simulink model "CustomSliders"  (R2025b)
settings: Solver=VariableStepAuto  StartTime=0.0  StopTime=10.0  RelTol=1e-3
settings Model: PacingRate=0.800000  Creator=The MathWorks, Inc.  LastModifiedBy=gkumares
settings OptimizationCC: ReuseModelBlockBuffer=off
settings RTWCC: GPUComputeCapability=3.5

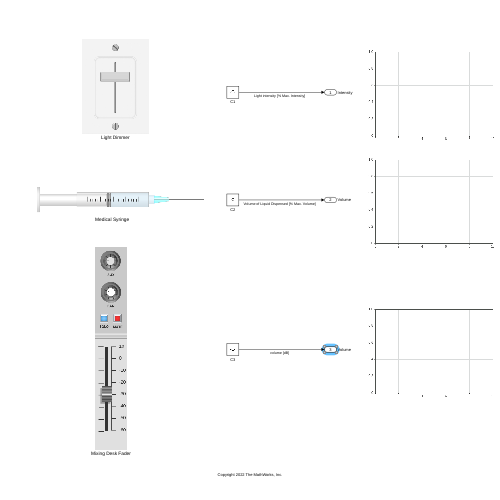
[thumbnail: Simulink's stored preview of the top-level diagram]
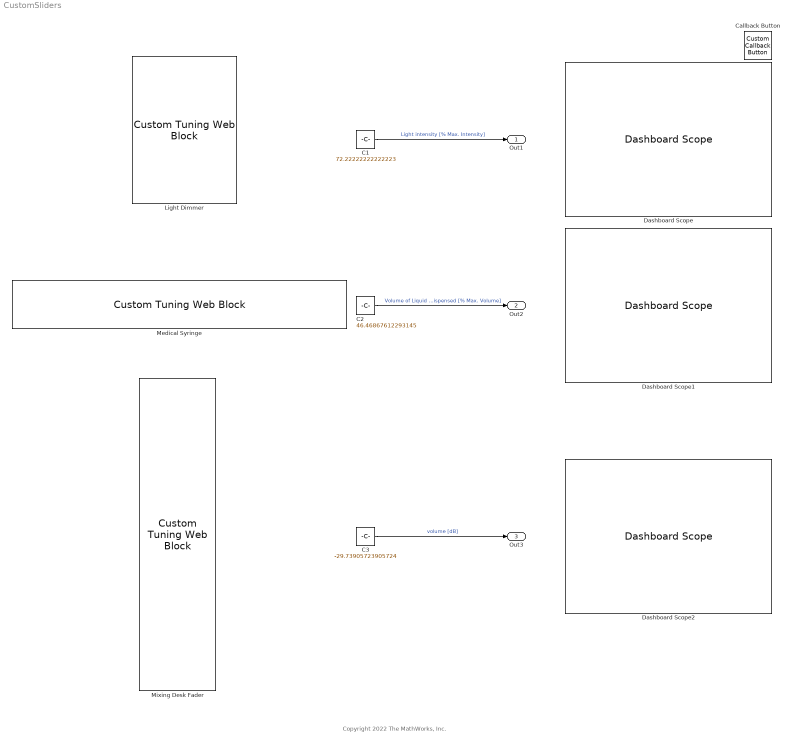
== system CustomSliders ==
  note: Copyright 2022 The MathWorks, Inc.
  C1 : Constant  Value=72.22222222222223
  C2 : Constant  Value=46.46867612293145
  C3 : Constant  Value=-29.73905723905724
  Callback Button : CustomCallbackButton  Configuration="{\"components\":[{\"name\":\"BackgroundImageComponent\",\"settings\":{\"image\":{\"size\":[0,0],\"src\":\"default\",\"srcOrientation\":\"Right\"},\"position\":[0,0,1,1]}},{\"name\":\"ButtonStateComponent\",\"settings\":{\"buttonType\":\"momentary\",\"clickFcn\":\"showExample('simulink\\/DesignCustomSlidersExample');\",\"onValue\":1,\"position\":[0,0,1,1],\"pressDelay\":\"500\",\"pressFcn\":\"\",\"repeatInterval\":\"0\",\"states\":[{\"horizontalAlignment\":\"center\",\"image\":{\"position\":[0,0,1,1],\"src\":\"default\",\"srcOrientation\":\"Right\"},\"label\":{\"color\":[0.01176470588,0.01176470588,0.01176470588,1],\"icon\":{\"size\":[0,0],\"src\":\"default\",\"srcOrientation\":\"Right\"},\"iconPlacement\":\"left\",\"text\":{\"content\":\"?\"}},\"labelOffset\":[0,0],\"verticalAlignment\":\"middle\"},{\"horizontalAlignment\":\"center\",\"image\":{\"position\":[0,0,1,1],\"src\":\"default\",\"srcOrientation\":\"Right\"},\"label\":{\"color\":[0.01176470588,0.01176470588,0.01176470588,1],\"icon\":{\"size\":[0,0],\"src\":\"default\",\"srcOrientation\":\"Right\"},\"iconPlacement\":\"left\",\"text\":{\"content\":\"?\"}},\"labelOffset\":[0,0],\"verticalAlignment\":\"middle\"},{\"horizontalAlignment\":\"center\",\"image\":{\"position\":[0,0,1,1],\"src\":\"default\",\"srcOrientation\":\"Right\"},\"label\":{\"color\":[0.01176470588,0.01176470588,0.01176470588,1],\"icon\":{\"size\":[0,0],\"src\":\"default\",\"srcOrientation\":\"Right\"},\"iconPlacement\":\"left\",\"text\":{\"content\":\"?\"}},\"labelOffset\":[0,0],\"verticalAlignment\":\"middle\"},{\"horizontalAlignment\":\"center\",\"image\":{\"position\":[0,0,1,1],\"src\":\"default\",\"srcOrientation\":\"Right\"},\"label\":{\"color\":[0.01176470588,0.01176470588,0.01176470588,1],\"icon\":{\"size\":[0,0],\"src\":\"default\",\"srcOrientation\":\"Right\"},\"iconPlacement\":\"left\",\"text\":{\"content\":\"?\"}},\"labelOffset\":[0,0],\"verticalAlignment\":\"middle\"}]}},{\"name\":\"ForegroundImageComponent\",\"settings\":{\"image\":{\"size\":[0,0],\"src\":\"default\",\"srcOrientation\":\"Right\"},\"isForeground\":1,\"position\":[0,0,1,1]}}],\"derived\":{\"blockParameters\":{\"AutoActivate\":true,\"ButtonText\":\"?\",\"ButtonType\":\"Momentary\",\"ClickFcn\":\"showExample('simulink\\/DesignCustomSlidersExample');\",\"OnValue\":1,\"PressDelay\":\"500\",\"PressFcn\":\"\",\"RepeatInterval\":\"0\",\"fixedAspectRatio\":\"off\"}},\"settings\":{\"BindingType\":\"standalone\",\"autoActivate\":true,\"backgroundColor\":[244,244,244,1],\"backgroundOffset\":0.2,\"backgroundOpacity\":1,\"fixedAspectRatio\":\"off\",\"foregroundColor\":[0.01176470588,0.01176470588,0.01176470588,1],\"migratedFromLegacy\":true,\"useBackgroundColor\":true,\"variant\":\"callback\",\"version\":\"R2025a\"},\"type\":\"Button\"}"  CustomBackgroundColor="{\"color\":[0.9568627451,0.9568627451,0.9568627451],\"show\":true}"
  Dashboard Scope : DashboardScope  Ymin=0  Ymax=1  FontColor=[0.0, 0.0, 0.0]
  Dashboard Scope1 : DashboardScope  Ymin=0  Ymax=1  FontColor=[0.0, 0.0, 0.0]
  Dashboard Scope2 : DashboardScope  Ymin=0  Ymax=1  FontColor=[0.0, 0.0, 0.0]
  Light Dimmer : CustomTuningWebBlock  LabelPosition=Hide  ShowInitialText=on  Configuration="{\"components\":[{\"name\":\"LinearScaleComponent\",\"settings\":{\"bounds\":{\"max\":100,\"min\":0,\"tickInterval\":\"auto\"},\"internalTickHeightScaleFactor\":0.5,\"labelColor\":[255,255,200],\"labelFont\":{\"font\":\"Arial\",\"fontSize\":12},\"labelOffset\":0.05,\"labelTransparency\":1,\"needleImage\":{\"size\":[1144,1604],\"src\":\"data:image\\/png;base64,iVBORw0KGgoAAAANSUhEUgAABHgAAAZECAYAAACZ1be8AAAAAXNSR0IArs4c6QAAAARnQU1BAACxjwv8YQUAAAAJcEhZcwAAMsAAADLAAShkWtsAADEiSURBVHhe7d35s9d13f\\/x\\/oGmbWqmnMpSy7AwM8usAM3UzA1cisIFM1EDAY0QBQ+LiiKCLFqAcBb2TZBN9gMKxL64gNLUKWumsn6pZrKpptfF83Wdz7mw8Opc+Xm\\/r4+H223mPhD1vX79fL6Pz+v9er8NAAAAAAAAAAAAAAAAAAAAAAAAAAAAAAAAAAAAAAAAAAAAAAAAAAAAAAAAAAAAAAAAAAAAAAAAAAAAAAAAAAAAAAAAAAAAAAAAAAAAAAAAAAAAAAAAAAAAAAAAAAAAAA ...(+16878 chars)\",\"srcOrientation\":\"Up\"},\"needleOffset\":[0.004661239495798319,-0.48886434750598196],\"needleSize\":{\"height\":1,\"width\":1},\"position\":[0.21691176470588236,0.44202098288238545,0.4734032762746181,0.5877100840336135],\"referencePoint\":\"auto\",\"scaleColors\":[],\"scaleColorsSize\":0.2,\"scaleDirection\":\"BT\",\"showLabels\":false,\"showMinorTicks\":0,\"showSpanLine\":false,\"showTicks\":false,\"tickColor\":[0,0,0],\"tickTransparency\":1,\"valueBarColor\":[0,114,189],\"valueBarOffset\":-0.27,\"valueBarSize\":0.1,\"valueBarTransparency\":0}},{\"name\":\"BackgroundImageComponent\",\"settings\":{\"image\":{\"size\":[1145,1605],\"src\":\"data:image\\/png;base64,iVBORw0KGgoAAAANSUhEUgAABHkAAAZFCAMAAACKlf8VAAAAAXNSR0IArs4c6QAAAARnQU1BAACxjwv8YQUAAAKUUExURdnZ2fLy8ubm5s3NzcHBwba2tqqqqp6enpKSkpGRkZqamqenp6WlpbKysq+vr729vbu7u8jIyOTk5Nra2q2traSkpKOjo6ampqioqKmpqaKiop+fn52dnZubm5iYmJOTk42NjYaGhri4uMXFxePj46ysrLCwsLOzs7Gxsa6urqurq6CgoJSUlI6OjsPDw6GhobS0tLW1tbe3t7m5ubq6upeXl4SEhImJieLi4ry8vL6+vr+\\/v8DAwIqKin9\\/f+Hh4cTExMLCwsbGxsfHx8nJycrKypycnJmZmZaWloKCgnNzc+Dg ...(+380064 chars)\",\"srcOrientation\":\"Up\"},\"position\":[0,0,1,1],\"scaleMode\":\"0\"}},{\"name\":\"ForegroundImageComponent\",\"settings\":{\"image\":{\"size\":[0,0],\"src\":\"default\",\"srcOrientation\":[]},\"isForeground\":1,\"position\":[0,0,1,1],\"scaleMode\":\"0\"}}],\"derived\":{\"blockParameters\":{\"ForegroundColor\":[0,0,0],\"Limits\":{\"Max\":100,\"Min\":0,\"Ticks\":\"auto\"},\"ScaleColors\":[],\"ScaleDirection\":\"Clockwise\",\"ScaleMax\":100,\"ScaleMin\":0,\"TickInterval\":\"auto\",\"fixedAspectRatio\":\"on\"}},\"settings\":{\"BindingType\":\"param\",\"aspectRatio\":3.7777777777777777,\"backgroundColor\":[0,0,0,\"1\"],\"backgroundOffset\":0,\"backgroundOpacity\":1,\"fixedAspectRatio\":\"on\",\"foregroundColor\":[252,252,196],\"orientation\":\"vertical\",\"showBackgroundColor\":false,\"value\":0,\"version\":\"R2023a\"},\"type\":\"LinearGauge\"}"
  Medical Syringe : CustomTuningWebBlock  LabelPosition=Hide  ShowInitialText=on  Configuration="{\"components\":[{\"name\":\"LinearScaleComponent\",\"settings\":{\"bounds\":{\"max\":100,\"min\":0,\"tickInterval\":\"auto\"},\"internalTickHeightScaleFactor\":0.5,\"labelColor\":[255,255,200],\"labelFont\":{\"font\":\"Arial\",\"fontSize\":12},\"labelOffset\":0.05,\"labelTransparency\":1,\"needleImage\":{\"size\":[2348,344],\"src\":\"data:image\\/png;base64,iVBORw0KGgoAAAANSUhEUgAACSwAAAFYCAMAAABk09DVAAAAAXNSR0IArs4c6QAAAARnQU1BAACxjwv8YQUAAAG\\/UExURQAAALbl\\/wAAAAQEBAcHBwgICAsLCwwMDA4ODhAQEBERERQUFBgYGBsbGx4eHh8fHyEhISMjIyQkJCYmJicnJykpKSoqKiwsLC0tLTAwMDMzMzY2Njc3Nzg4ODo6Ojs7Oz09PUBAQEJCQkNDQ0VFRUZGRkdHR0lJSUtLS0xMTE5OTlBQUFFRUVJSUlNTU1RUVFZWVlhYWFlZWVpaWltbW11dXV9fX2FhYWJiYmNjY2RkZGZmZmdnZ2lpaWpqamtra2xsbG1tbW5ubm9vb3BwcHFxcXJycnNzc3R0dHV1dXZ2dnd3 ...(+5320 chars)\",\"srcOrientation\":\"Right\"},\"needleOffset\":[-0.10051546391752578,-0.004172421731123388],\"needleSize\":{\"height\":1,\"width\":1},\"position\":[0.01885680612846199,0.3773020257826888,0.26033034069981587,0.973089766254174],\"referencePoint\":\"auto\",\"scaleColors\":[],\"scaleColorsSize\":0.2,\"scaleDirection\":\"LR\",\"showLabels\":false,\"showMinorTicks\":0,\"showSpanLine\":false,\"showTicks\":false,\"tickColor\":[0,0,0],\"tickTransparency\":1,\"valueBarColor\":[0,114,189],\"valueBarOffset\":-0.27,\"valueBarSize\":0.1,\"valueBarTransparency\":0}},{\"name\":\"BackgroundImageComponent\",\"settings\":{\"image\":{\"size\":[2348,344],\"src\":\"data:image\\/png;base64,iVBORw0KGgoAAAANSUhEUgAACSwAAAFYCAMAAABk09DVAAAAAXNSR0IArs4c6QAAAARnQU1BAACxjwv8YQUAAAAGUExURf\\/\\/\\/wAAAFXC034AAAACdFJOU\\/8A5bcwSgAAAAlwSFlzAAAywAAAMsABKGRa2wAAAyVJREFUeF7twQEBAAAAgiD\\/r25IQAAAAAAAAAAAAAAAAAAAAAAAAAAAAAAAAAAAAAAAAAAAAAAAAAAAAAAAAAAAAAAAAAAAAAAAAAAAAAAAAAAAAAAAAAAAAAAAAAAAAAAAAAAAAAAAAAAAAAAAAAAAAAAAAAAAAAAAAAAAAAAAAAAAAAAAAAAAAAAAAAAAAAAAAAAAAAAAAAAAAAAAAAAAAAAAAAAAAAAAAAAAAAAAAAAAAAAAAAAAAAAAAAAAAAAAAAAAAAAAAAAAAAAAAAAAAAAAAAAAAAAAAAAAAAAAAAAAAAAAAAAAAAAAAAAAAAAAAAAAAAAAAAAAAAAAAAAAAAAAAAAAAAAAAAAAAAAAAAAAAAAAAAAAAAAAAAAAAAAAAAAAAAAAAAAAAAAAAAAAAAAAAAAAAAAAAAAAAAAAAAAAAAAAAAAAAAAAAAAAAAAAAAAAAAAAAAAAAAAAAAAAAAAAAAAAAAAAAAAAAAAAAAAAAAAAAAAAAAAAAAAAAAAAAAAAAAAAAAAAAAAAAAAAAAAAAAAAAAAAAAAAAAAAAAAAAAAAAAAAAAAAAAAAAAAAAAAAAAAAAAAAAAAAAAAAAAAAAAAAAAAAAAAAAAAAAAAAAAAAAAAAAAAAAAAAAAAAAAAAAAAAAAAAAAAAAAAAAAAAAAAAAAAAAAAAAAAAAAAAAAAAAAAAAAAAAAAAAAAAAAAAAAAAAAAAAAAAAAAAAAAAAAAAAAAAAAAAAAAAAAAAAAAAAAAAAAAAAAAAAAAAAAAAAAAAAAAAAAAAAAAAAAAAAAAAAAAAAAAAAAAAAAAAAAAAAAAAAAAAAAAAAAAAAAAAAAAAAAAAAAAAAAAAAAAAAAAAAAAAAAAAAAAAAAAAAAAAAAAAAAAAAAAAAAAAAAAAAAAAAAAAAAAAAAAAAAAAAAAAAAAAAAAAAAAAAAAAAAAAAAAAAAAAAAAAAAAAAAAAAAAAAAAAAAAAAAAAAAAAAAAAAAAAAAAAAAAAAAAAAAAAAAAAAAAAAAAAAAAAAAAAAAAAAAAAAAAAAAAAAAAAAAAAAAAAAAAAAAAAAAAAwLkaVSwAAQ05s70AAAAASUVORK5CYII=\",\"srcOrientation\":\"Right\"},\"position\":[0,0,1,1],\"scaleMode\":\"0\"}},{\"name\":\"ForegroundImageComponent\",\"settings\":{\"angle\":0,\"image\":{\"size\":[2348,344],\"src\":\"data:image\\/png;base64,iVBORw0KGgoAAAANSUhEUgAACSwAAAFYCAYAAABTDSDnAAAAAXNSR0IArs4c6QAAAARnQU1BAACxjwv8YQUAAAAJcEhZcwAAMsAAADLAAShkWtsAADmMSURBVHhe7d3Lr271nef3Uv8LPahRS51ZR1EPMkikTNKtZJRJRVYGUalqUKNuKRlE6o6UKBXZD5wrHC7masAGcylsc\\/EFMBgHzB0frjZ3MMdwDBjDMcXdGOOjvX95nu31xe3sjx9Xzm9vs9Zer5f0lqqsr89X+FmDtc7vV66\\/AAAAAAAAAAAAAAAAAAAAAAAAAAAAAAAAAAAAAAAAAAAAAAAAAAAAAAAAAAAAAAAAAAAAAAAAAAAAAAAAAAAAAAAAAAAAAAAAAAAAAAAAAAAAAAAA ...(+20020 chars)\"},\"isForeground\":1,\"position\":[0,0.0017840699815837937,1,1],\"scaleMode\":\"0\"}}],\"derived\":{\"blockParameters\":{\"ForegroundColor\":[0,0,0],\"Limits\":{\"Max\":100,\"Min\":0,\"Ticks\":\"auto\"},\"ScaleColors\":[],\"ScaleDirection\":\"Clockwise\",\"ScaleMax\":100,\"ScaleMin\":0,\"TickInterval\":\"auto\",\"fixedAspectRatio\":\"on\"}},\"settings\":{\"BindingType\":\"param\",\"aspectRatio\":3.7777777777777777,\"backgroundColor\":[0,0,0,\"1\"],\"backgroundOffset\":0,\"backgroundOpacity\":1,\"fixedAspectRatio\":\"on\",\"foregroundColor\":[252,252,196],\"orientation\":\"horizontal\",\"showBackgroundColor\":false,\"value\":0,\"version\":\"R2023a\"},\"type\":\"LinearGauge\"}"
  Mixing Desk Fader : CustomTuningWebBlock  LabelPosition=Hide  ShowInitialText=on  Configuration="{\"components\":[{\"name\":\"LinearScaleComponent\",\"settings\":{\"bounds\":{\"max\":10,\"min\":-60,\"tickInterval\":\"auto\"},\"internalTickHeightScaleFactor\":1,\"labelColor\":[0,0,0],\"labelFont\":{\"font\":\"Arial\",\"fontSize\":12},\"labelOffset\":0.15,\"labelTransparency\":1,\"needleImage\":{\"size\":[97,144],\"src\":\"data:image\\/png;base64,iVBORw0KGgoAAAANSUhEUgAAAGEAAACQCAMAAAAvFvUtAAAAAXNSR0IArs4c6QAAAARnQU1BAACxjwv8YQUAAAGDUExURQAAAAAAAAAAAAAAAAAAAAAAAAAAAAAAAAAAAAAAAAAAAAAAAAAAAAAAAAAAAAAAAAAAAAAAAAAAAAAAAAAAAAAAAAAAAAAAAAAAAAAAAAAAAAAAAAAAAAAAAAAAAAAAAAAAAAAAAAAAAAAAAAAAAAAAAAAAAAAAAAAAAAAAAAAAAAAAAAAAAAAAAAAAAAAAAAAAAAAAAAAAAAAAAAAAAAAAAAAAAAAAAAAAAAAAAAAAAAAAAAAAAAAAAAAAAAAAAAAAAAAAAAAAAAAAAAAAAAAAAAAAAAAAAAsLCw8PDxQUFBUVFRgYGBwcHB0dHR4eHiIiIicnJysrKywsLC0tLS8vLzMzMzY2Njc3Nzo6Ojw8PD4+Pj8\\/P0BAQEJCQkREREdHR0hISElJSUxMTE1NTVBQUFNTU1RUVFZWVldXV1hYWFlZWV1dXV5eXl9fX2FhYWJiYmZmZmdnZ2hoaG1tbXJycnNzc3Z2dnd3d3h4eHl5eXp6ent7e319fX5+fn9\\/f\\/\\/\\/\\/6No\\/zUAAABIdFJOUwABAgMEBQYHCQoLDA0PEBETFBUWFxgZHh8gJCUmJygpKi0uMDU2Nzg5Ojs8PT5DRUhJSktMTU9QU1RXWFlaW1xdX2BiY2RlZiW8Jv8AAAAJcEhZcwAAMsAAADLAAShkWtsAAANjSURBVGhD7dvnUxpRFMZhdpeVFVERRCMasMREBUsUNTZUUNJ7Lze9997bnx5gD3iXvB+c8VVmHJ+vzvAb3fWcu+Pq+5\\/ikk\\/VqeNMsHCGCRYuMMHCVSZYuM0ECw+ZYOEpk1swPNRrpnLBMEzT2qDeMZUKpmUHnGBTlfrIVCwYlu2EWtoi0Qr1mUkVf0S209rR1ZNI9gr1jalYMAOhju7+Q8Pp9KhL\\/WQqFZyWff3D44czmWmX+s1ULFjBtu6D40fms9lll\\/rDVCo0RfYPT8xncxXqF1O5EE2mM9nc+nrBpb4w6QUJFNQHpmphOVcoHHWx5xIo3GSChXNMsMCFCmeZYOEaEyzI\\/uOAhVdMsCC7gwMWvjLBgswsjjoVZGZxwMItJljgQoXTTLBwhQkW7jLBwgsmWHjPBAufmGDhBxMsyHmQAxa+M8HCWyZYuM4EC1z1KchJhwMW5KTDAQty0uGABTnpcMCCnHQ4YEFOOhywIOcQjjoV5KTDoRU2nkXlpMOhF6rP01yVgv7E\\/pdpZwsS2K6Cfi\\/J1zj2Cpuxawtc5UJvelovyA7nkMKopyA7nAN+D7LDOeB1kB3OAQuywzlgQXY4ByzIhuWoU0F2OAcsyA7ngAWuHSrsirnkLchE4YAFmSgc8DrIROFwCzX3kkwUDliQ33eOOhVkonDAgkwUjmpBP3tzaYXtfwaSQEGdZPJcB6HOM8GCzCwOT6FyL91hgoVHTLDwnAkWZO5ywMIbJlh4yQQLD5iqBf13+hKTXtjBuXSMyXMdhDrBBAtyWuPwFCr3kkxFDli4zAQL8q4fByzcYIIFeZuQAxbuMcGCTBQOWJDtxAELT5hgQd5t4oAF2bAcsCB\\/u+aAhWdMsPCYCRbuM8GCTBQOWLjIBAunmGCBCxS2olDILU+P9kabLKP0jnTZXqHWXmEz6laIJFNTS6tr6wxrq0uZdDJSW0iMTC6u5PNrW5fPryxOphLeghkMxw+Mzc4tLDIszM2ODcbDQVMvOK1dA6mJqZlZhpmpidRAV6ujF4xAKBbvGxwaSTGMDA32xWOhgLFR8Bm20xLrjPckOHrinbEWx9YCPp9lNzaHo+2xDoZYezTc3Ghb8tkuw\\/Q3BJyixq0rfUygwa9dhTLDtPw2j9+qDZTJf+owyCe6fL5\\/r11ccaKXahgAAAAASUVORK5CYII=\",\"srcOrientation\":\"Up\"},\"needleOffset\":[0.08688981868898187,-0.987981765437215],\"needleSize\":{\"height\":0.08821358267716535,\"width\":0.24522357723577234},\"position\":[0.46776574803149606,0.4168346774193548,0.4002016129032258,0.4586921751968504],\"referencePoint\":\"auto\",\"scaleColors\":[],\"scaleColorsSize\":0.2,\"scaleDirection\":\"BT\",\"showLabels\":1,\"showMinorTicks\":0,\"showSpanLine\":1,\"showTicks\":1,\"tickColor\":[0,0,0],\"tickTransparency\":1,\"valueBarColor\":[0,114,189],\"valueBarOffset\":-0.27,\"valueBarSize\":0.1,\"valueBarTransparency\":0}},{\"name\":\"BackgroundImageComponent\",\"settings\":{\"image\":{\"size\":[406,1651],\"src\":\"data:image\\/png;base64,iVBORw0KGgoAAAANSUhEUgAAAZYAAAZzCAYAAADY1hEpAAAAAXNSR0IArs4c6QAAAARnQU1BAACxjwv8YQUAAAAJcEhZcwAAMsAAADLAAShkWtsAAMnjSURBVHhe7b0J2GxZWZ6NgChODIqgIMjUIJOMMiMiiCLiPIM0QzM18zxDN4OMCt3QdCNT093QdDMLiHEekiBRcYyiRhM1ahKHJCbmz\\/8n1v89dc57ep11nlW1dn3rPaeq9v1c133B+WrXfndVrV53rbX23nUlQgghZGgW5IT880E++9nPLgAAVqG+4mi3QYoglkZ+9md\\/FgBgJcQHsTTiGhEAQAnxQSyNuEYEAFBCfBBLI64RAQCUEB\\/E0ohrRAAAJcQHsTTiGhEAQAnxQSyNuE ...(+70622 chars)\",\"srcOrientation\":\"Up\"},\"position\":[0,0,1,1],\"scaleMode\":\"0\"}},{\"name\":\"ForegroundImageComponent\",\"settings\":{\"image\":{\"size\":[0,0],\"src\":\"default\",\"srcOrientation\":[]},\"isForeground\":1,\"position\":[0,0,1,1],\"scaleMode\":\"0\"}}],\"derived\":{\"blockParameters\":{\"ForegroundColor\":[0,0,0],\"Limits\":{\"Max\":10,\"Min\":-60,\"Ticks\":\"auto\"},\"ScaleColors\":[],\"ScaleDirection\":\"Clockwise\",\"ScaleMax\":10,\"ScaleMin\":-60,\"TickInterval\":\"auto\",\"fixedAspectRatio\":\"on\"}},\"settings\":{\"BindingType\":\"param\",\"aspectRatio\":3.7777777777777777,\"backgroundColor\":[0,0,0,\"1\"],\"backgroundOffset\":0,\"backgroundOpacity\":1,\"fixedAspectRatio\":\"on\",\"foregroundColor\":[252,252,196],\"orientation\":\"vertical\",\"showBackgroundColor\":false,\"value\":0,\"version\":\"R2023a\"},\"type\":\"LinearGauge\"}"
  Out1 : Outport  SignalName=Intensity
  Out2 : Outport  Port=2  SignalName=Volume
  Out3 : Outport  Port=3  SignalName=Volume
  wires:
  C1/1 -> Out1/1  "Light intensity [% Max. Intensity]"
  C2/1 -> Out2/1  "Volume of Liquid Dispensed [% Max. Volume]"
  C3/1 -> Out3/1  "volume [dB]"
